simulink model "HR_old"  (R2022a)
settings: Solver=FixedStepDiscrete  StartTime=0.0  StopTime=10.0  FixedStep=0.04  RelTol=1e-3
PreLoadFcn:
  | listing = dir;
  | if (contains([listing .name], 'AGR')) && (contains([listing .name], 'MAP'))
  |     addpath('./AGR', './MAP');
  |     addpath( genpath('./MAP') );
  | elseif (contains([listing .name], 'HR.slx'))
  |     addpath('../AGR', '../MAP');
  |     addpath( genpath('../MAP') );
  | else
  | 
  | end
  | 
  | load('BusStructureHR.mat');
InitFcn:
  | listing = dir;
  | if (contains([listing .name], 'AGR')) && (contains([listing .name], 'MAP'))
  |     addpath('./AGR', './MAP');
  |     addpath( genpath('./MAP') );
  | elseif (contains([listing .name], 'HR.slx'))
  |     addpath('../AGR', '../MAP');
  |     addpath( genpath('../MAP') );
  | else
  | 
  | end
  | 
  | load('BusStructureHR.mat');
StartFcn:
  | listing = dir;
  | if (contains([listing .name], 'AGR')) && (contains([listing .name], 'MAP'))
  |     addpath('./AGR', './MAP');
  |     addpath( genpath('./MAP') );
  | elseif (contains([listing .name], 'HR.slx'))
  |     addpath('../AGR', '../MAP');
  |     addpath( genpath('../MAP') );
  | else
  | 
  | end
  | 
  | load('BusStructureHR.mat');
undefined symbols (not defined in the file): HRDataTagWrap, HRElevationValid, HRImpactPointElevation, HRSelected, HRSelectedWraparound, HRTargetOffMap, HRTargetRangeEast, HRTargetRangeNorth, llh, ne, ned2ECEF, pECEF_ip, pECEF_ref
settings Model: Creator=ASCL  LastModifiedBy=ASCL
settings SolverCC: AlgebraicLoopSolver=TrustRegion
settings DataIOCC: SaveOutput=off  SignalLogging=off  DSMLogging=off  SaveTime=off  ReturnWorkspaceOutputs=off
settings OptimizationCC: DefaultParameterBehavior=Inlined  UseDivisionForNetSlopeComputation=on  GainParamInheritBuiltInType=on  UseFloatMulNetSlope=on  InlineInvariantSignals=on  BufferReuse=off  ExpressionFolding=off  PassReuseOutputArgsAs=Individual arguments  ZeroExternalMemoryAtStartup=off  ZeroInternalMemoryAtStartup=off  NoFixptDivByZeroProtection=on  LifeSpan=1  OptimizeBlockOrder=speed  DifferentSizesBufferReuse=on
settings DebuggingCC: ParameterTunabilityLossMsg=error  UnconnectedInputMsg=warning  UnconnectedOutputMsg=warning  UnconnectedLineMsg=warning  SFMachineParentedDataDiag=warning  ArithmeticOperatorsInVariantConditions=warning
settings HardwareCC: ProdBitPerPointer=32  ProdBitPerSizeT=32  ProdBitPerPtrDiffT=32  ProdLargestAtomicInteger=Long  ProdLargestAtomicFloat=Double  ProdEndianess=BigEndian  ProdWordSize=32  ProdLongLongMode=on  ProdHWDeviceType=Freescale->MPC83xx
settings ModelReferenceCC: ModelReferenceNumInstancesAllowed=Single
settings SFSimCC: SimUserLibraries=MAPd.lib WS2_32.lib  SimUseLocalCustomCode=off  MATLABDynamicMemAlloc=off  CustomCodeUndefinedFunction=UseInterfaceOnly
settings SFSimCC: SimCustomHeaderCode=|
  | #include "MAP.h"
  | #include "MAPDATA.h"
  | #include "DVOF.h"
  | #include "userDefined.h"
settings SFSimCC: SimUserSources=|
  | MAP.c
  | DVOF.c
  | userDefined.c
settings RTWCC: SystemTargetFile=ert.tlc  TemplateMakefile=ert_default_tmf  GenerateReport=on  RTWUseLocalCustomCode=off  RTWUseSimCustomCode=on  CustomLibrary=MAPd.lib WS2_32.lib  IncludeHyperlinkInReport=on  LaunchReport=on  GenerateTraceInfo=on  GenerateTraceReport=on  GenerateTraceReportSl=on  GenerateTraceReportSf=on  GenerateTraceReportEml=on  GenerateCodeMetricsReport=on
settings RTWCC: CustomHeaderCode=|
  | #include "MAP.h"
  | #include "MAPDATA.h"
  | #include "DVOF.h"
  | #include "userDefined.h"
settings RTWCC: CustomSource=|
  | MAP.c
  | DVOF.c
  | userDefined.c
settings CodeAppCC: ForceParamTrailComments=on  IgnoreCustomStorageClasses=off  OperatorAnnotations=on  SimulinkDataObjDesc=on  SFDataObjDesc=on  CustomSymbolStrUtil=HR_$N$C  InsertBlockDesc=on  EnableCustomComments=on
settings ERTTargetCC: TargetLangStandard=C99 (ISO)  UtilityFuncGeneration=Shared location  GenerateSampleERTMain=on  IncludeMdlTerminateFcn=off  CombineSignalStateStructs=on  SuppressErrorStatus=on  SupportAbsoluteTime=off  SupportComplex=off  InlinedParameterPlacement=NonHierarchical  ERTCustomFileTemplate=example_file_process.tlc  ERTFilePackagingFormat=CompactWithDataFile  EnableSignedLeftShifts=off  EnableSignedRightShifts=off

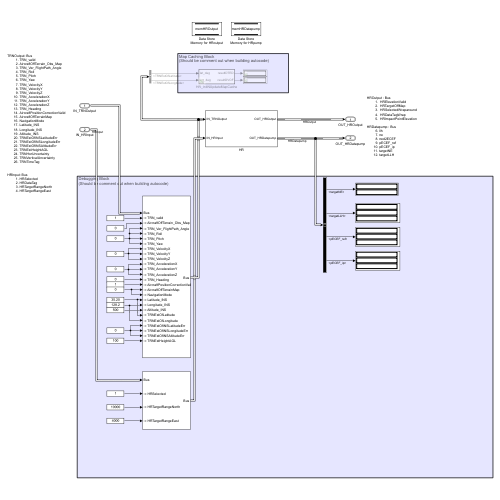
[thumbnail: Simulink's stored preview of the top-level diagram]
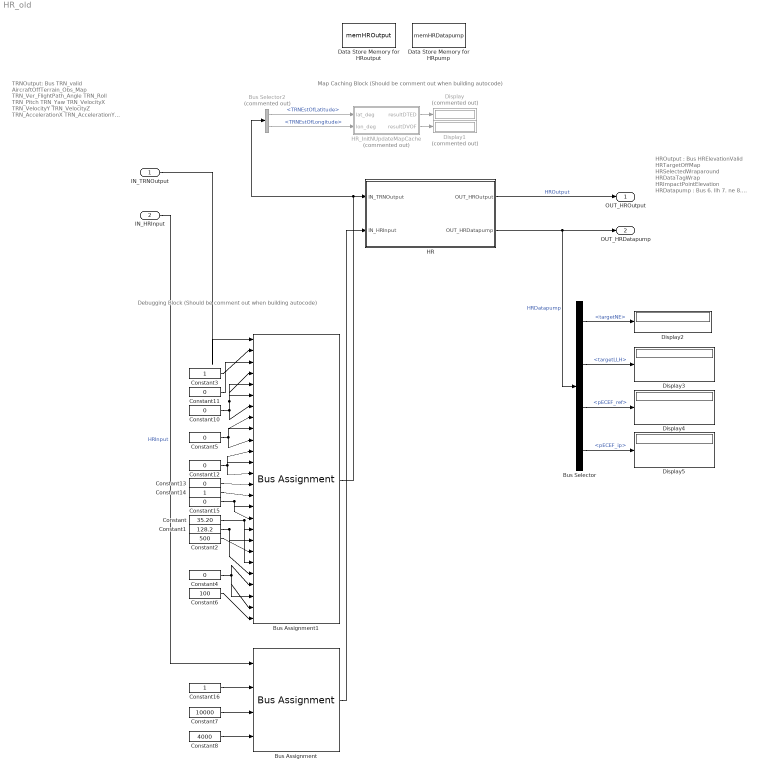
== system HR_old ==
  note: TRNOutput: Bus
      | TRN_valid
      | AircraftOffTerrain_Obs_Map
      | TRN_Ver_FlightPath_Angle
      | TRN_Roll
      | TRN_Pitch
      | TRN_Yaw
      | TRN_VelocityX
      | TRN_VelocityY
      | TRN_VelocityZ
      | TRN_AccelerationX
      | TRN_AccelerationY
      | TRN_AccelerationZ
      | TRN_Heading
      | AircraftPositionCorrectionValid
      | AircraftOffTerrainMap
      | NavigationMode
      | Latitude_INS
      | Longitude_INS
      | Altitude_INS
      | TRNEstOfINSLatitudeErr
      | TRNEstOfINSLongitudeErr
      | TRNEstOfINSAltitudeErr
      | TRNEstHeightAGL
      | TRNHorUncertainty
      | TRNVerticalUncertainty
      | TRNTimeTag
      |
      | HRInput: Bus
      | HRSelected
      | HRDataTag
      | HRTargetRangeNorth
      | HRTargetRangeEast
  note: HROutput : Bus
      | HRElevationValid
      | HRTargetOffMap
      | HRSelectedWraparound
      | HRDataTagWrap
      | HRImpactPointElevation
      |
      | HRDatapump : Bus
      | 6. llh
      | 7. ne
      | 8. ned2ECEF
      | 9. pECEF_ref
      | 10. pECEF_ip
      | 11. targetNE
      | 12. targetLLH
  note: Map Caching Block
      | (Should be comment out when building autocode)
  note: Debugging Block
      | (Should be comment out when building autocode)
  IN_TRNOutput : Inport  OutDataTypeStr=Bus: TRNOutput  BusOutputAsStruct=on
  IN_HRInput : Inport  Port=2  OutDataTypeStr=Bus: HRInput  BusOutputAsStruct=on
  Bus Assignment : BusAssignment  AssignedSignals=HRSelected,HRTargetRangeNorth,HRTargetRangeEast
  Bus Assignment1 : BusAssignment  AssignedSignals=TRN_valid,AircraftOffTerrain_Obs_Map,TRN_Ver_FlightPath_Angle,TRN_Roll,TRN_Pitch,TRN_Yaw,TRN_VelocityX,TRN_VelocityY,TRN_VelocityZ,TRN_AccelerationX,TRN_AccelerationY,TRN_AccelerationZ,TRN_Heading,AircraftPositionCorrectionValid,AircraftOffTerrainMap,NavigationMode,Latitude_INS,Longitude_INS,Altitude_INS,TRNEstOfLatitude,TRNEstOfLongitude,TRNEstOfINSLatitudeErr,TRNEstOfINSLongitudeErr,TRNEstOfINSAltitudeErr,TRNEstHeightAGL
  Bus Selector : BusSelector  OutputSignals=targetNE,targetLLH,pECEF_ref,pECEF_ip
  Bus Selector2 : BusSelector  Commented=on  OutputSignals=TRNEstOfLatitude,TRNEstOfLongitude
  Constant : Constant  Value=35.20
  Constant1 : Constant  Value=128.2
  Constant{4..5,10,12..13} (5 alike) : Constant  Value=0
  Constant11 : Constant  Value=0  OutDataTypeStr=boolean
  Constant14 : Constant  OutDataTypeStr=boolean
  Constant15 : Constant  Value=0  OutDataTypeStr=boolean
  Constant16 : Constant  OutDataTypeStr=boolean
  Constant2 : Constant  Value=500
  Constant3 : Constant  OutDataTypeStr=boolean
  Constant6 : Constant  Value=100  OutDataTypeStr=uint16
  Constant7 : Constant  Value=10000  OutDataTypeStr=double
  Constant8 : Constant  Value=4000  OutDataTypeStr=double
  Data Store Memory for HRoutput : DataStoreMemory  DataStoreName=memHROutput  ReadBeforeWriteMsg=warning  WriteAfterWriteMsg=warning  WriteAfterReadMsg=warning  VectorParams1D=off  ShowAdditionalParam=off  OutDataTypeStr=Bus: HROutput
  Data Store Memory for HRpump : DataStoreMemory  DataStoreName=memHRDatapump  ReadBeforeWriteMsg=warning  WriteAfterWriteMsg=warning  WriteAfterReadMsg=warning  VectorParams1D=off  ShowAdditionalParam=off  OutDataTypeStr=Bus: HRDatapump
  Display : Display  Commented=on
  Display1 : Display  Commented=on
  Display{2..5} (4 alike) : Display
  HR : Subsystem
      mask init:
      | % latGPS = double(0);
      | % lonGPS = double(0);
      | % altGPS = double(0);
      | % velEGPS = double(0);
      | % velNGPS = double(0);
      | % velUGPS = double(0);
      | % notValidGPS = boolean(0);
      | % notAvaildINS = boolean(0);
      | % velUINS = double(0);
      | % velVINS = double(0);
      | % velWINS = double(0);
      | % rollINS = double(0);
      | % pitchINS = double(0);
      | % hgdINS = double(0);
      | % accXINS = double(0);
      | % accYINS = double(0);
      | % accZINS = double(0);
      | % activated = boolean(0);
      | % reactionT = uint16(0);
      | % pullUpG = uint16(0);
      | % rollRate = uint16(0);
      | % gOnsetRate = uint16(0);
      | % maxGamma = uint16(0);
      | % setWarnH = double(0);
      | % obsWarningTime = uint16(1);
      | % wiresWarningTime = uint16(1);
      | % latErrOfINS = double(0);
      | % lonErrOfINS = double(0);
      | % altErrorofINS = uint16(0);
      | % heightEstOfTRN = uint16(0);
      | % horUncertaintyOfTRN = double(0);
      | % verUncertaintyOfTRN = double(0);
  HR_InitNUpdateMapCache : Subsystem  Commented=on  TreatAsAtomicUnit=on
  OUT_HROutput : Outport  OutDataTypeStr=Bus: HROutput  VectorParamsAs1DForOutWhenUnconnected=off  BusOutputAsStruct=on
  OUT_HRDatapump : Outport  Port=2  OutDataTypeStr=Bus: HRDatapump  VectorParamsAs1DForOutWhenUnconnected=off  BusOutputAsStruct=on
  wires:
  IN_HRInput/1 -> Bus Assignment/1  "HRInput"
  HR/2(OUT_HRDatapump) -> Bus Selector/1, OUT_HRDatapump/1  "HRDatapump"
  HR/1(OUT_HROutput) -> OUT_HROutput/1  "HROutput"
  HR_InitNUpdateMapCache/2(resultDVOF) -> Display1/1
  HR_InitNUpdateMapCache/1(resultDTED) -> Display/1
  Bus Selector/1 -> Display2/1  "<targetNE>"
  Bus Selector/2 -> Display3/1  "<targetLLH>"
  Bus Selector/4 -> Display5/1  "<pECEF_ip>"
  Bus Selector/3 -> Display4/1  "<pECEF_ref>"
  Constant10/1 -> Bus Assignment1/7, Bus Assignment1/4, Bus Assignment1/5, Bus Assignment1/6
  Constant5/1 -> Bus Assignment1/10, Bus Assignment1/8, Bus Assignment1/9
  Constant12/1 -> Bus Assignment1/13, Bus Assignment1/11, Bus Assignment1/12
  Constant6/1 -> Bus Assignment1/26
  Constant15/1 -> Bus Assignment1/17, Bus Assignment1/16
  Constant13/1 -> Bus Assignment1/14
  Constant4/1 -> Bus Assignment1/23, Bus Assignment1/25, Bus Assignment1/24
  Constant11/1 -> Bus Assignment1/3
  Constant14/1 -> Bus Assignment1/15
  Constant/1 -> Bus Assignment1/21, Bus Assignment1/18
  Constant3/1 -> Bus Assignment1/2
  Constant1/1 -> Bus Assignment1/22, Bus Assignment1/19
  Constant2/1 -> Bus Assignment1/20
  IN_TRNOutput/1 -> Bus Assignment1/1
  Bus Assignment/1 -> HR/2(IN_HRInput)
  Constant16/1 -> Bus Assignment/2
  Constant7/1 -> Bus Assignment/3
  Constant8/1 -> Bus Assignment/4
  Bus Assignment1/1 -> HR/1(IN_TRNOutput), Bus Selector2/1
  Bus Selector2/2 -> HR_InitNUpdateMapCache/2(lon_deg)  "<TRNEstOfLongitude>"
  Bus Selector2/1 -> HR_InitNUpdateMapCache/1(lat_deg)  "<TRNEstOfLatitude>"

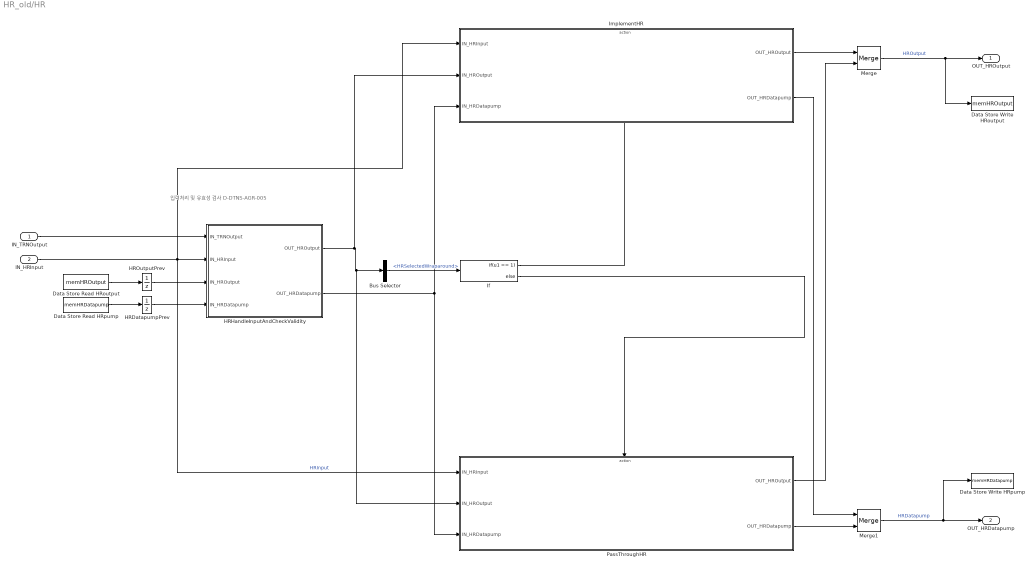
== system HR_old/HR ==
  note: 입력처리 및 유효성 검사 D-DTNS-AGR-005
  IN_TRNOutput : Inport  OutDataTypeStr=Bus: TRNOutput
  IN_HRInput : Inport  Port=2  OutDataTypeStr=Bus: HRInput
  Bus Selector : BusSelector  OutputSignals=HRSelectedWraparound
  Data Store Read HRoutput : DataStoreRead  DataStoreName=memHROutput  IndexOptions=Index vector (dialog)  Indices=1  OutputSizes=1
  Data Store Read HRpump : DataStoreRead  DataStoreName=memHRDatapump  IndexOptions=Index vector (dialog)  Indices=1  OutputSizes=1
  Data Store Write HRoutput : DataStoreWrite  DataStoreName=memHROutput  IndexOptions=Index vector (dialog)  Indices=1  OutputSizes=1
  Data Store Write HRpump : DataStoreWrite  DataStoreName=memHRDatapump  IndexOptions=Index vector (dialog)  Indices=1  OutputSizes=1
  HRDatapumpPrev : UnitDelay  SampleTime=-1  HasFrameUpgradeWarning=on
  HRHandleInputAndCheckValidity : Subsystem  TreatAsAtomicUnit=on
      settings: RTWSystemCode=Nonreusable function  RTWFcnNameOpts=Use subsystem name
  HROutputPrev : UnitDelay  SampleTime=-1  HasFrameUpgradeWarning=on
  If : If  IfExpression=u1 == 1
  ImplementHR : Subsystem  TreatAsAtomicUnit=on
      settings: RTWSystemCode=Nonreusable function  RTWFcnNameOpts=Use subsystem name
  Merge : Merge
  Merge1 : Merge
  PassThroughHR : Subsystem  TreatAsAtomicUnit=on
      settings: RTWSystemCode=Nonreusable function  RTWFcnNameOpts=Use subsystem name
  OUT_HROutput : Outport  OutDataTypeStr=Bus: HROutput  VectorParamsAs1DForOutWhenUnconnected=off
  OUT_HRDatapump : Outport  Port=2  OutDataTypeStr=Bus: HRDatapump  VectorParamsAs1DForOutWhenUnconnected=off
  wires:
  Merge/1 -> Data Store Write HRoutput/1, OUT_HROutput/1  "HROutput"
  Merge1/1 -> Data Store Write HRpump/1, OUT_HRDatapump/1  "HRDatapump"
  If/1 -> ImplementHR/Action
  If/2 -> PassThroughHR/Action
  Data Store Read HRoutput/1 -> HROutputPrev/1
  IN_HRInput/1 -> ImplementHR/1(IN_HRInput), PassThroughHR/1(IN_HRInput), HRHandleInputAndCheckValidity/2(IN_HRInput)  "HRInput"
  Data Store Read HRpump/1 -> HRDatapumpPrev/1
  HRHandleInputAndCheckValidity/1(OUT_HROutput) -> ImplementHR/2(IN_HROutput), PassThroughHR/2(IN_HROutput), Bus Selector/1
  Bus Selector/1 -> If/1  "<HRSelectedWraparound>"
  HRHandleInputAndCheckValidity/2(OUT_HRDatapump) -> PassThroughHR/3(IN_HRDatapump), ImplementHR/3(IN_HRDatapump)
  ImplementHR/1(OUT_HROutput) -> Merge/1
  PassThroughHR/2(OUT_HRDatapump) -> Merge1/2
  PassThroughHR/1(OUT_HROutput) -> Merge/2
  ImplementHR/2(OUT_HRDatapump) -> Merge1/1
  IN_TRNOutput/1 -> HRHandleInputAndCheckValidity/1(IN_TRNOutput)
  HROutputPrev/1 -> HRHandleInputAndCheckValidity/3(IN_HROutput)
  HRDatapumpPrev/1 -> HRHandleInputAndCheckValidity/4(IN_HRDatapump)

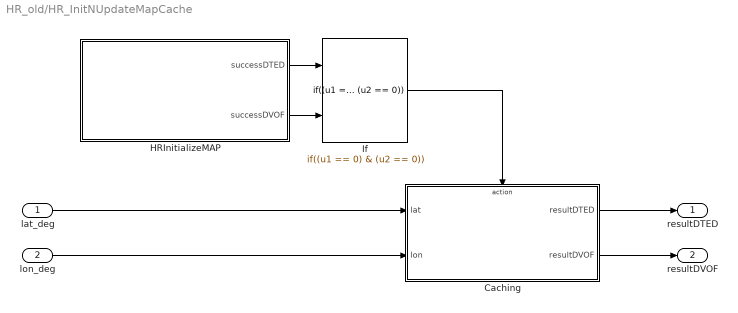
== system HR_old/HR_InitNUpdateMapCache ==
  lat_deg : Inport
  lon_deg : Inport  Port=2
  Caching : Subsystem  TreatAsAtomicUnit=on
  HRInitializeMAP : MATLAB Function  TreatAsAtomicUnit=on
  If : If  NumInputs=2  IfExpression=(u1 == 0) & (u2 == 0)  ShowElse=off
  resultDTED : Outport  VectorParamsAs1DForOutWhenUnconnected=off
  resultDVOF : Outport  Port=2  VectorParamsAs1DForOutWhenUnconnected=off
  wires:
  Caching/1(resultDTED) -> resultDTED/1
  HRInitializeMAP/1(successDTED) -> If/1
  Caching/2(resultDVOF) -> resultDVOF/1
  HRInitializeMAP/2(successDVOF) -> If/2
  If/1 -> Caching/Action
  lat_deg/1 -> Caching/1(lat)
  lon_deg/1 -> Caching/2(lon)

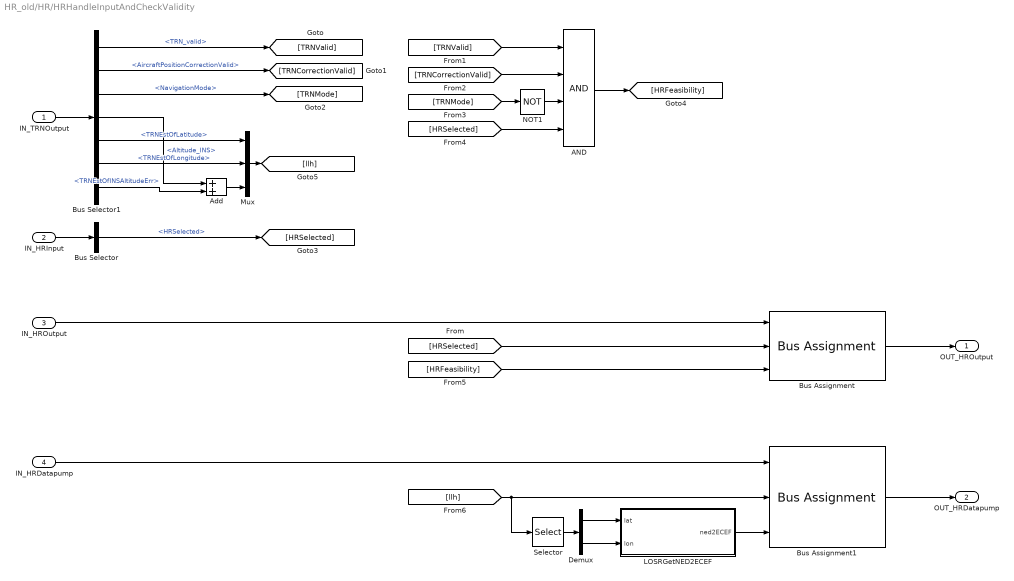
== system HR_old/HR/HRHandleInputAndCheckValidity ==
  IN_TRNOutput : Inport  OutDataTypeStr=Bus: TRNOutput
  IN_HRInput : Inport  Port=2  OutDataTypeStr=Bus: HRInput
  IN_HROutput : Inport  Port=3  OutDataTypeStr=Bus: HROutput
  IN_HRDatapump : Inport  Port=4  OutDataTypeStr=Bus: HRDatapump
  AND : Logic  Inputs=4  AllPortsSameDT=off  OutDataTypeStr=boolean
  Add : Sum
  Bus Assignment : BusAssignment  AssignedSignals=HRSelectedWraparound,HRElevationValid
  Bus Assignment1 : BusAssignment  AssignedSignals=llh,ned2ECEF
  Bus Selector : BusSelector  OutputSignals=HRSelected
  Bus Selector1 : BusSelector  OutputSignals=TRN_valid,AircraftPositionCorrectionValid,NavigationMode,Altitude_INS,TRNEstOfLatitude,TRNEstOfLongitude,TRNEstOfINSAltitudeErr
  Demux : Demux  Outputs=2
  LOSRGetNED2ECEF : MATLAB Function  TreatAsAtomicUnit=on
  Mux : Mux  Inputs=3
  NOT1 : Logic  Operator=NOT  IconShape=distinctive  AllPortsSameDT=off  OutDataTypeStr=boolean
  Selector : Selector  InputPortWidth=3  IndexOptions=Index vector (dialog)  Indices=[1 2]  OutputSizes=1
  OUT_HROutput : Outport  OutDataTypeStr=Bus: HROutput  VectorParamsAs1DForOutWhenUnconnected=off
  OUT_HRDatapump : Outport  Port=2  OutDataTypeStr=Bus: HRDatapump  VectorParamsAs1DForOutWhenUnconnected=off
  wires:
  IN_HRInput/1 -> Bus Selector/1
  IN_HROutput/1 -> Bus Assignment/1
  Bus Assignment/1 -> OUT_HROutput/1
  IN_HRDatapump/1 -> Bus Assignment1/1
  Bus Selector/1 -> [HRSelected]  "<HRSelected>"
  IN_TRNOutput/1 -> Bus Selector1/1
  Bus Selector1/5 -> Mux/1  "<TRNEstOfLatitude>"
  Bus Selector1/2 -> [TRNCorrectionValid]  "<AircraftPositionCorrectionValid>"
  Add/1 -> Mux/3
  Bus Selector1/1 -> [TRNValid]  "<TRN_valid>"
  Mux/1 -> [llh]
  Bus Selector1/6 -> Mux/2  "<TRNEstOfLongitude>"
  Bus Selector1/3 -> [TRNMode]  "<NavigationMode>"
  Bus Selector1/7 -> Add/2  "<TRNEstOfINSAltitudeErr>"
  Bus Selector1/4 -> Add/1  "<Altitude_INS>"
  [HRSelected] -> Bus Assignment/2
  [TRNValid] -> AND/1
  AND/1 -> [HRFeasibility]
  [TRNCorrectionValid] -> AND/2
  [HRSelected] -> AND/4
  NOT1/1 -> AND/3
  [TRNMode] -> NOT1/1
  [HRFeasibility] -> Bus Assignment/3
  Bus Assignment1/1 -> OUT_HRDatapump/1
  Selector/1 -> Demux/1
  Demux/2 -> LOSRGetNED2ECEF/2(lon)
  LOSRGetNED2ECEF/1(ned2ECEF) -> Bus Assignment1/3
  Demux/1 -> LOSRGetNED2ECEF/1(lat)
  [llh] -> Selector/1, Bus Assignment1/2

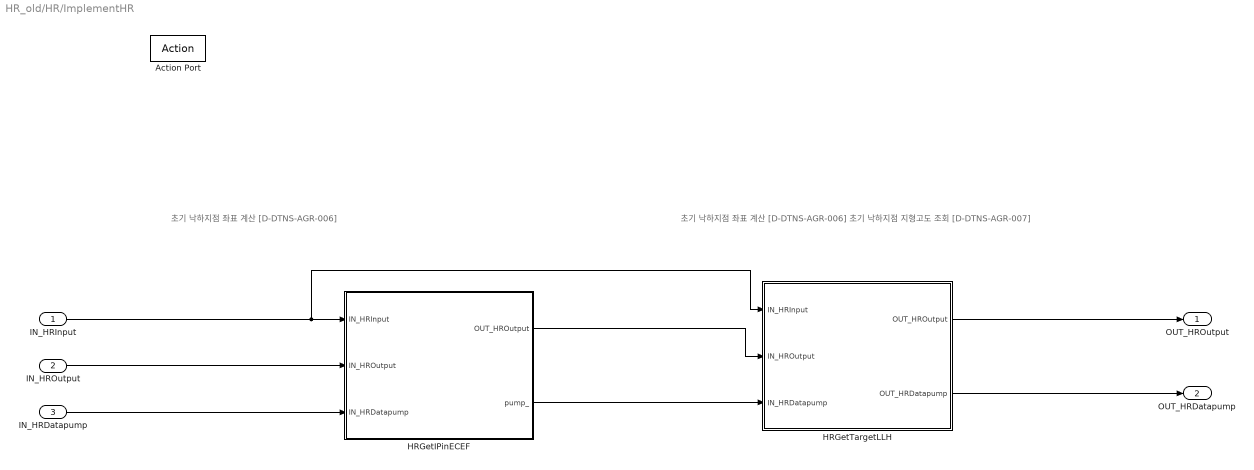
== system HR_old/HR/ImplementHR ==
  note: 초기 낙하지점 좌표 계산 [D-DTNS-AGR-006]
  note: 초기 낙하지점 좌표 계산 [D-DTNS-AGR-006]
      | 초기 낙하지점 지형고도 조회 [D-DTNS-AGR-007]
  IN_HRInput : Inport  OutDataTypeStr=Bus: HRInput
  IN_HROutput : Inport  Port=2  OutDataTypeStr=Bus: HROutput
  IN_HRDatapump : Inport  Port=3  OutDataTypeStr=Bus: HRDatapump
  Action Port : ActionPort  ActionPortLabel=if(u1 == 1)
  HRGetIPinECEF : Subsystem  TreatAsAtomicUnit=on
      settings: RTWSystemCode=Nonreusable function  RTWFcnNameOpts=Use subsystem name
  HRGetTargetLLH : Subsystem  TreatAsAtomicUnit=on
      settings: RTWSystemCode=Nonreusable function  RTWFcnNameOpts=Use subsystem name
  OUT_HROutput : Outport  OutDataTypeStr=Bus: HROutput  VectorParamsAs1DForOutWhenUnconnected=off
  OUT_HRDatapump : Outport  Port=2  OutDataTypeStr=Bus: HRDatapump  VectorParamsAs1DForOutWhenUnconnected=off
  wires:
  HRGetIPinECEF/1(OUT_HROutput) -> HRGetTargetLLH/2(IN_HROutput)
  HRGetIPinECEF/2(pump_) -> HRGetTargetLLH/3(IN_HRDatapump)
  IN_HRDatapump/1 -> HRGetIPinECEF/3(IN_HRDatapump)
  HRGetTargetLLH/1(OUT_HROutput) -> OUT_HROutput/1
  HRGetTargetLLH/2(OUT_HRDatapump) -> OUT_HRDatapump/1
  IN_HRInput/1 -> HRGetTargetLLH/1(IN_HRInput), HRGetIPinECEF/1(IN_HRInput)
  IN_HROutput/1 -> HRGetIPinECEF/2(IN_HROutput)

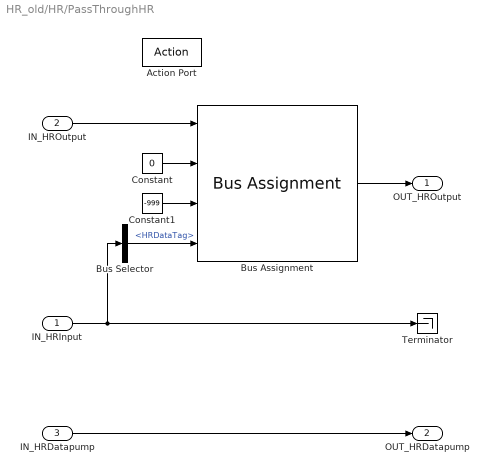
== system HR_old/HR/PassThroughHR ==
  IN_HRInput : Inport  OutDataTypeStr=Bus: HRInput
  IN_HROutput : Inport  Port=2  OutDataTypeStr=Bus: HROutput
  IN_HRDatapump : Inport  Port=3  OutDataTypeStr=Bus: HRDatapump
  Action Port : ActionPort  ActionPortLabel=else
  Bus Assignment : BusAssignment  AssignedSignals=HRElevationValid,HRImpactPointElevation,HRDataTagWrap
  Bus Selector : BusSelector  OutputSignals=HRDataTag
  Constant : Constant  Value=0  OutDataTypeStr=boolean
  Constant1 : Constant  Value=-999  OutDataTypeStr=int16
  Terminator : Terminator
  OUT_HROutput : Outport  OutDataTypeStr=Bus: HROutput  VectorParamsAs1DForOutWhenUnconnected=off
  OUT_HRDatapump : Outport  Port=2  OutDataTypeStr=Bus: HRDatapump  VectorParamsAs1DForOutWhenUnconnected=off
  wires:
  IN_HROutput/1 -> Bus Assignment/1
  Bus Assignment/1 -> OUT_HROutput/1
  IN_HRDatapump/1 -> OUT_HRDatapump/1
  Constant/1 -> Bus Assignment/2
  IN_HRInput/1 -> Bus Selector/1, Terminator/1
  Bus Selector/1 -> Bus Assignment/4  "<HRDataTag>"
  Constant1/1 -> Bus Assignment/3

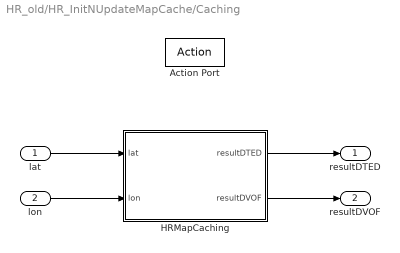
== system HR_old/HR_InitNUpdateMapCache/Caching ==
  lat : Inport
  lon : Inport  Port=2
  Action Port : ActionPort  ActionPortLabel=if((u1 == 0) & (u2 == 0))
  HRMapCaching : MATLAB Function  TreatAsAtomicUnit=on
  resultDTED : Outport  VectorParamsAs1DForOutWhenUnconnected=off
  resultDVOF : Outport  Port=2  VectorParamsAs1DForOutWhenUnconnected=off
  wires:
  HRMapCaching/1(resultDTED) -> resultDTED/1
  lat/1 -> HRMapCaching/1(lat)
  lon/1 -> HRMapCaching/2(lon)
  HRMapCaching/2(resultDVOF) -> resultDVOF/1

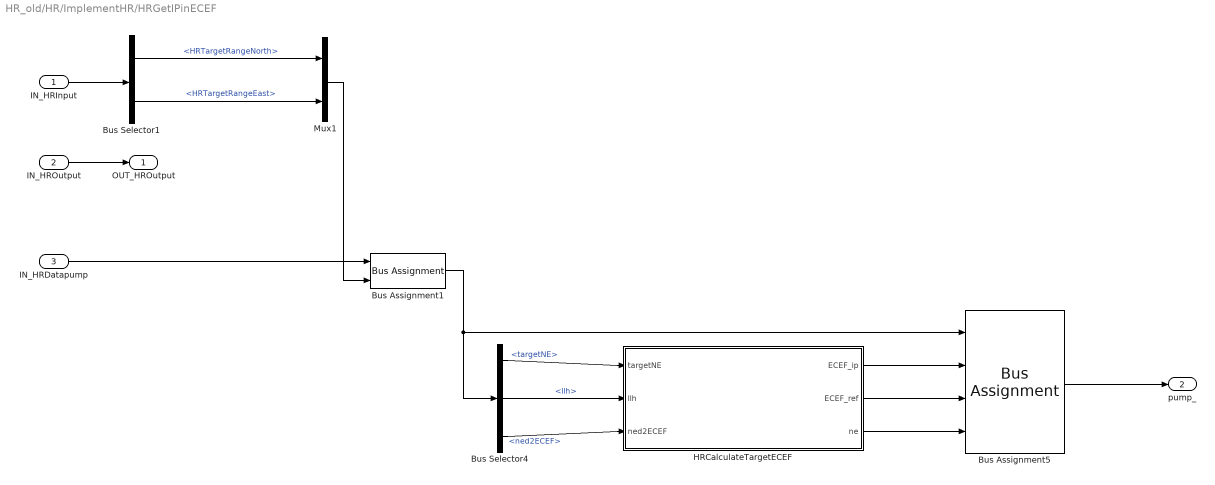
== system HR_old/HR/ImplementHR/HRGetIPinECEF ==
  IN_HRInput : Inport  OutDataTypeStr=Bus: HRInput
  IN_HROutput : Inport  Port=2  OutDataTypeStr=Bus: HROutput
  IN_HRDatapump : Inport  Port=3  OutDataTypeStr=Bus: HRDatapump
  Bus Assignment1 : BusAssignment  AssignedSignals=targetNE
  Bus Assignment5 : BusAssignment  AssignedSignals=pECEF_ip,pECEF_ref,ne
  Bus Selector1 : BusSelector  OutputSignals=HRTargetRangeNorth,HRTargetRangeEast
  Bus Selector4 : BusSelector  OutputSignals=targetNE,llh,ned2ECEF
  HRCalculateTargetECEF : MATLAB Function  TreatAsAtomicUnit=on
  Mux1 : Mux  Inputs=2
  OUT_HROutput : Outport  OutDataTypeStr=Bus: HROutput  VectorParamsAs1DForOutWhenUnconnected=off
  pump_ : Outport  Port=2  OutDataTypeStr=Bus: HRDatapump  VectorParamsAs1DForOutWhenUnconnected=off
  wires:
  IN_HRInput/1 -> Bus Selector1/1
  IN_HROutput/1 -> OUT_HROutput/1
  IN_HRDatapump/1 -> Bus Assignment1/1
  Bus Selector1/1 -> Mux1/1  "<HRTargetRangeNorth>"
  Bus Selector1/2 -> Mux1/2  "<HRTargetRangeEast>"
  Mux1/1 -> Bus Assignment1/2
  Bus Assignment1/1 -> Bus Selector4/1, Bus Assignment5/1
  Bus Assignment5/1 -> pump_/1
  Bus Selector4/1 -> HRCalculateTargetECEF/1(targetNE)  "<targetNE>"
  Bus Selector4/2 -> HRCalculateTargetECEF/2(llh)  "<llh>"
  Bus Selector4/3 -> HRCalculateTargetECEF/3(ned2ECEF)  "<ned2ECEF>"
  HRCalculateTargetECEF/3(ne) -> Bus Assignment5/4
  HRCalculateTargetECEF/2(ECEF_ref) -> Bus Assignment5/3
  HRCalculateTargetECEF/1(ECEF_ip) -> Bus Assignment5/2

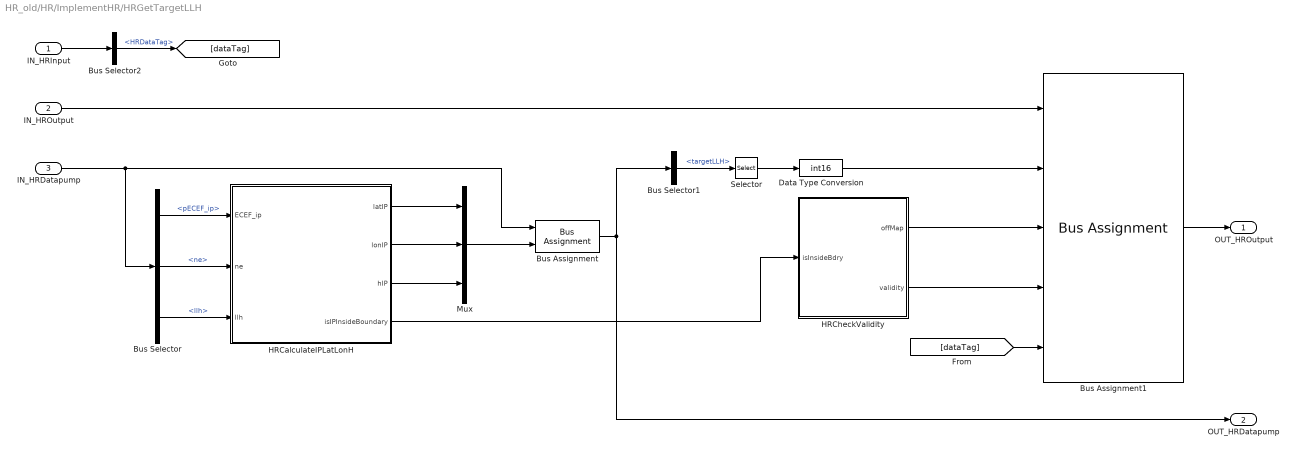
== system HR_old/HR/ImplementHR/HRGetTargetLLH ==
  IN_HRInput : Inport  OutDataTypeStr=Bus: HRInput
  IN_HROutput : Inport  Port=2  OutDataTypeStr=Bus: HROutput
  IN_HRDatapump : Inport  Port=3  OutDataTypeStr=Bus: HRDatapump
  Bus Assignment : BusAssignment  AssignedSignals=targetLLH
  Bus Assignment1 : BusAssignment  AssignedSignals=HRImpactPointElevation,HRTargetOffMap,HRElevationValid,HRDataTagWrap
  Bus Selector : BusSelector  OutputSignals=pECEF_ip,ne,llh
  Bus Selector1 : BusSelector  OutputSignals=targetLLH
  Bus Selector2 : BusSelector  OutputSignals=HRDataTag
  Data Type Conversion : DataTypeConversion  OutDataTypeStr=int16  SaturateOnIntegerOverflow=off  RndMeth=Floor
  HRCalculateIPLatLonH : MATLAB Function  TreatAsAtomicUnit=on
  HRCheckValidity : MATLAB Function  TreatAsAtomicUnit=on
  Mux : Mux  Inputs=3
  Selector : Selector  IndexMode=Zero-based  InputPortWidth=3  IndexOptions=Index vector (dialog)  Indices=2  OutputSizes=1
  OUT_HROutput : Outport  OutDataTypeStr=Bus: HROutput  VectorParamsAs1DForOutWhenUnconnected=off
  OUT_HRDatapump : Outport  Port=2  OutDataTypeStr=Bus: HRDatapump  VectorParamsAs1DForOutWhenUnconnected=off
  wires:
  IN_HRInput/1 -> Bus Selector2/1
  Bus Assignment/1 -> Bus Selector1/1, OUT_HRDatapump/1
  IN_HROutput/1 -> Bus Assignment1/1
  IN_HRDatapump/1 -> Bus Assignment/1, Bus Selector/1
  Mux/1 -> Bus Assignment/2
  Bus Assignment1/1 -> OUT_HROutput/1
  Bus Selector1/1 -> Selector/1  "<targetLLH>"
  Selector/1 -> Data Type Conversion/1
  Data Type Conversion/1 -> Bus Assignment1/2
  HRCalculateIPLatLonH/1(latIP) -> Mux/1
  HRCalculateIPLatLonH/2(lonIP) -> Mux/2
  HRCalculateIPLatLonH/3(hIP) -> Mux/3
  Bus Selector/1 -> HRCalculateIPLatLonH/1(ECEF_ip)  "<pECEF_ip>"
  Bus Selector/2 -> HRCalculateIPLatLonH/2(ne)  "<ne>"
  Bus Selector2/1 -> [dataTag]  "<HRDataTag>"
  [dataTag] -> Bus Assignment1/5
  HRCalculateIPLatLonH/4(isIPInsideBoundary) -> HRCheckValidity/1(isInsideBdry)
  HRCheckValidity/1(offMap) -> Bus Assignment1/3
  HRCheckValidity/2(validity) -> Bus Assignment1/4
  Bus Selector/3 -> HRCalculateIPLatLonH/3(llh)  "<llh>"

== matlab function HR_old/HR/ImplementHR/HRGetTargetLLH/HRCheckValidity ==
  data: isInsideBdry input; offMap output; validity output
function [offMap, validity] = HRCheckValidity(isInsideBdry)

offMap = false;
validity = true;

if isInsideBdry == 1
    offMap = false;
    validity = true;
else
    offMap = true;
    validity = false;
end

== matlab function HR_old/HR/ImplementHR/HRGetIPinECEF/HRCalculateTargetECEF ==
  data: targetNE input; ECEF_ip output; llh input; ned2ECEF input; ECEF_ref output; ne output
function [ECEF_ip, ECEF_ref, ne] = HRCalculateTargetECEF(targetNE, llh, ned2ECEF)

% Initialization
ECEF_ip = zeros(1,3);
ECEF_ref = zeros(1,3);
ne = 0.0;

% Define constants
R_Ea            = 6378137.0;        % Earth semi-major axis [m]
e               = 0.08181919;       % Earth eccentricity

lat = llh(1);
lon = llh(2);
alt = llh(3);

% Get the prime vertical radius of curvature, N_{E} = ne
ne = R_Ea / sqrt(1 - e^2*(sind(lat))^2 );

% Calculate ECEF Coordinates of the current vehicle position as reference
ECEF_ref(1) = (ne + alt) * cosd(lat) * cosd(lon);
ECEF_ref(2) = (ne + alt) * cosd(lat) * sind(lon);
ECEF_ref(3) = (ne * (1 - e^2) + alt) * sind(lat); 

% Calculate ECEF Coordinates of the impact point
pNED = [targetNE(1), targetNE(2), alt];

ECEF_ip(1) = ned2ECEF(1)*pNED(1) + ned2ECEF(2)*pNED(2) + ned2ECEF(3)*pNED(3) + ECEF_ref(1);
ECEF_ip(2) = ned2ECEF(4)*pNED(1) + ned2ECEF(5)*pNED(2) + ned2ECEF(6)*pNED(3) + ECEF_ref(2);
ECEF_ip(3) = ned2ECEF(7)*pNED(1) + ned2ECEF(8)*pNED(2) + ned2ECEF(9)*pNED(3) + ECEF_ref(3);

== matlab function HR_old/HR_InitNUpdateMapCache/HRInitializeMAP ==
  data: successDTED output; successDVOF output
function [successDTED, successDVOF] = HRInitializeMAP()

flagDTED = int32(1);
flagDVOF = int32(1);

pathDTED = 'C:\Users\ASCL\Documents\GitHub\DTNS\MAP\MAP_DB\';
pathDVOF = 'C:\Users\ASCL\Documents\GitHub\DTNS\MAP\DVOF\';

strLenDTED = int32(strlength(pathDTED));
strLenDVOF = int32(strlength(pathDVOF));

flagDTED = coder.ceval('InitialMap', pathDTED, strLenDTED );
flagDVOF = coder.ceval('InitDVOF', pathDVOF, strLenDVOF );

successDTED = flagDTED;
successDVOF = flagDVOF;

== matlab function HR_old/HR_InitNUpdateMapCache/Caching/HRMapCaching ==
  data: resultDTED output; resultDVOF output; lat input; lon input
function [resultDTED, resultDVOF] = HRMapCaching(lat, lon)

resultDTED = int32(1);
resultDVOF = int32(1);

resultDVOF = coder.ceval('UpdateObstList', lat, lon);
resultDTED = coder.ceval('UpdateMapCache', lat, lon);

== matlab function HR_old/HR/ImplementHR/HRGetTargetLLH/HRCalculateIPLatLonH ==
  data: ECEF_ip input; latIP output; ne input; llh input; lonIP output; hIP output; isIPInsideBoundary output
function [latIP, lonIP, hIP, isIPInsideBoundary] = HRCalculateIPLatLonH(ECEF_ip, ne, llh)

latIP = 0.0;
lonIP = 0.0;
hIP = 0.0;
alt = llh(3);

isIPInsideBoundary = int32(0);

% Define constants
e               = 0.08181919;       % Earth eccentricity

% Calcuate Geodetic Coordinates of Impact Points using ECEF Coordinates
latIP = asind( ECEF_ip(3) / (ne * (1 - e^2) ));
lonIP = atan2d( ECEF_ip(2), ECEF_ip(1) );

% Check if Target is Off Map
isIPInsideBoundary = coder.ceval('IsScanBoundary', latIP, lonIP);
% isIPInsideBoundary = int32(1);

% Get Target Height
hIP = coder.ceval('GetElevation', latIP, lonIP);

== matlab function HR_old/HR/HRHandleInputAndCheckValidity/LOSRGetNED2ECEF ==
  data: lat input; ned2ECEF output; lon input
function ned2ECEF = LOSRGetNED2ECEF(lat, lon)
%LOSRGetNED2ECEF Compute transformation matrix from local NED to ECEF frame
% Input
% lat       : Current aircraft latitude [deg]
% lon       : Current aircraft longitude [deg]
% Output
% ned2ECEF  : Rotation matrix in single 1D array form
% *Note : (ECEF Vecotr) = (ned2ECEF) * (NED Vector) + (ECEF, Reference)

% Initialize
ned2ECEF = zeros(1,9);

% NED to ECEF Transformation Matrix
ned2ECEF(1,1) = -sind(lat)*cosd(lon);
ned2ECEF(1,2) = -sind(lon);
ned2ECEF(1,3) = -cosd(lat)*cosd(lon);

ned2ECEF(1,4) = -sind(lat)*sind(lon);
ned2ECEF(1,5) = cosd(lon);
ned2ECEF(1,6) = -cosd(lat)*sind(lon);

ned2ECEF(1,7) = cosd(lat);
ned2ECEF(1,8) = 0.0;
ned2ECEF(1,9) = -sind(lat);

end
